simulink library "mttlib"  (R2022a)
settings: Solver=VariableStepAuto  StartTime=0.0  StopTime=10.0  RelTol=1e-3
libraries: etargetslib x5, simulink x3, instrumentseriallib x3
settings Model: Creator=chrismailer  LastModifiedBy=chrismailer

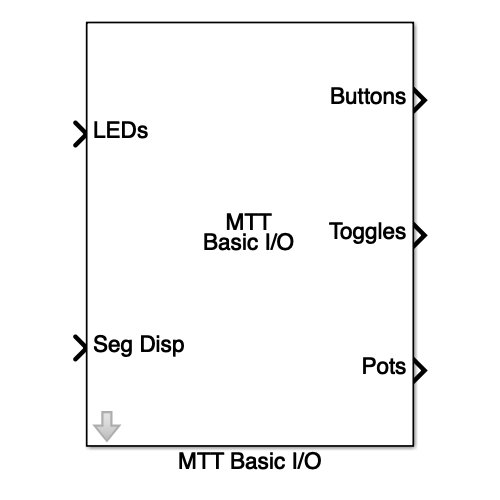
[thumbnail: Simulink's stored preview of the top-level diagram]
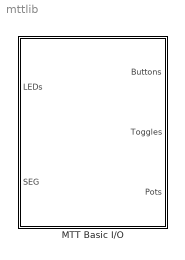
== system mttlib ==
  MTT Basic I/O : Subsystem  mask{SelectedPort=/dev/cu.BLTH, SampleTime=0.01}
      mask prompts: SelectedPort "Port:"; SampleTime "Sample Time:"
      mask help: Configure the parameters for communicating with the MTT.
      mask init:
      | % update popup with serial ports
      |     mask = Simulink.Mask.get(gcb);
      |     param = mask.getParameter('SelectedPort');
      |     param.TypeOptions = ['<Select a port...>', serialportlist];
      |     % configure port of serial blocks
      |     set_param([gcb '/Serial Configuration'],'Port',SelectedPort)
      |     set_param([gcb '/Serial Send'],'Port',SelectedPort)
      |     set_param([gcb '/Serial Receive'],'Port',SelectedPort)
      |     set_param([gcb '/Serial Receive'],'SampleTime',num2str(SampleTime))
      mask TypeOptions SelectedPort: <Select a port...> | /dev/cu.BLTH | /dev/tty.BLTH | /dev/cu.Bluetooth-Incoming-Port | /dev/tty.Bluetooth-Incoming-Port
      mask Display:
      | disp('MTT\nBasic I/O');
      | port_label('output', 1, 'Buttons');
      | port_label('output', 2, 'Toggles');
      | port_label('output', 3, 'Pots');
      | port_label('input', 1, 'LEDs');
      | port_label('input', 2, 'Seg Disp');

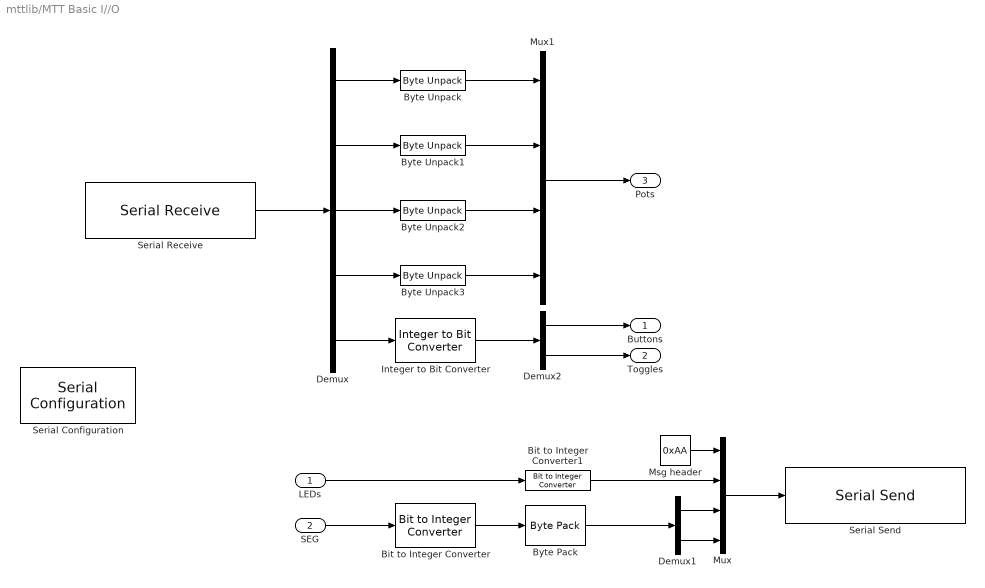
== system mttlib/MTT Basic I//O ==
  LEDs : Inport  OutDataTypeStr=boolean
  SEG : Inport  Port=2  OutDataTypeStr=boolean
  Bit to Integer Converter : simulink/Logic and Bit Operations/Bit to Integer Converter  nbits=11  bitOrder=MSB first  signedOutputValues=Unsigned  outDtype=uint16  outDtypeSigned=Inherit via internal rule
      settings: SourceProductBaseCode=SL
  Bit to Integer Converter1 : simulink/Logic and Bit Operations/Bit to Integer Converter  nbits=8  bitOrder=MSB first  signedOutputValues=Unsigned  outDtype=uint8  outDtypeSigned=Inherit via internal rule
      settings: SourceProductBaseCode=SL
  Byte Pack : etargetslib/Byte Pack  datatypes={'uint16'}  byteAlign=1
  Byte Unpack{,1..3} (4 alike) : etargetslib/Byte Unpack  dimensions={[1]}  datatypes={'uint16'}  byteAlign=1
  Demux : Demux  Outputs=[2,2,2,2,1]
  Demux1 : Demux  Outputs=2
  Demux2 : Demux  Outputs=2
  Integer to Bit Converter : simulink/Logic and Bit Operations/Integer to Bit Converter  nbits=8  signedInputValues=Unsigned  bitOrder=MSB first  outDtype=boolean
      settings: SourceProductBaseCode=SL
  Msg header : Constant  Value=0xAA
  Mux : Mux
  Mux1 : Mux
  Serial Configuration : instrumentseriallib/Serial Configuration  Priority=-200000  PortSel=/dev/cu.BLTH  Port=/dev/cu.BLTH  ComPort=/dev/cu.BLTH  BaudRate=115200  DataBits=8  Parity=none  StopBits=1  ByteOrder=little-endian  FlowControl=none  Timeout=10  SimulateUsing=Interpreted execution  BlockInModel=on  aMode=1
      settings: SourceProductBaseCode=OT,IC,MT
  Serial Receive : instrumentseriallib/Serial Receive  Priority=1  PortSel=/dev/cu.BLTH  Port=/dev/cu.BLTH  ComPort=/dev/cu.BLTH  DataType=uint8  SaveDataType=uint8  ToggleHeader=on  Header=[0xAA]  ToggleTerminator=off  Terminator=<none>  CustomTerminator=[]  InputFormat=Column major  ToggleDataSize=on  DataSize=[1 9]  EnableBlockingMode=on  ActionDataUnavailable=Output last received value  ActionWhenDataUnavailable=Output last received value  CustomValue=0  SampleTime=0.01  SimulateUsing=Interpreted execution  BlockInModel=on  aMode=1
      settings: SourceProductBaseCode=OT,IC,MT
  Serial Send : instrumentseriallib/Serial Send  Priority=1  PortSel=/dev/cu.BLTH  Port=/dev/cu.BLTH  ComPort=/dev/cu.BLTH  Header=[]  Terminator=<none>  CustomTerminator=[]  EnableBlockingMode=on  SimulateUsing=Interpreted execution  BlockInModel=on  aMode=1
      settings: SourceProductBaseCode=OT,IC,MT
  Buttons : Outport
  Toggles : Outport  Port=2
  Pots : Outport  Port=3  OutDataTypeStr=uint16
  wires:
  Demux1/2 -> Mux/4
  Byte Unpack1/1 -> Mux1/2
  Demux/2 -> Byte Unpack1/1
  Msg header/1 -> Mux/1
  Demux1/1 -> Mux/3
  Byte Unpack/1 -> Mux1/1
  Demux/1 -> Byte Unpack/1
  Demux/3 -> Byte Unpack2/1
  Mux/1 -> Serial Send/1
  Demux/4 -> Byte Unpack3/1
  Serial Receive/1 -> Demux/1
  Demux/5 -> Integer to Bit Converter/1
  Byte Unpack2/1 -> Mux1/3
  Byte Unpack3/1 -> Mux1/4
  Integer to Bit Converter/1 -> Demux2/1
  Demux2/1 -> Buttons/1
  Demux2/2 -> Toggles/1
  LEDs/1 -> Bit to Integer Converter1/1
  Mux1/1 -> Pots/1
  Bit to Integer Converter1/1 -> Mux/2
  SEG/1 -> Bit to Integer Converter/1
  Byte Pack/1 -> Demux1/1
  Bit to Integer Converter/1 -> Byte Pack/1
